simulink model "func2_b"  (R2020a)
settings: Solver=VariableStepAuto  StartTime=0.0  StopTime=10.0  RelTol=1e-3  EnableMultiTasking=on
undefined symbols (not defined in the file or in its folder): S, vsva2197, xcvc1902
libraries: ModelComposer x2, parametrization_2_lib x1
settings Model: Creator=abehbood  LastModifiedBy=viswanad
settings DataIOCC: ReturnWorkspaceOutputs=off
settings OptimizationCC: LifeSpan=inf
settings DebuggingCC: SFUnexpectedBacktrackingDiag=warning  SFNoUnconditionalDefaultTransitionDiag=warning  ArithmeticOperatorsInVariantConditions=warning
settings SFSimCC: SimUseLocalCustomCode=off  CustomCodeUndefinedFunction=UseInterfaceOnly
settings RTWCC: RTWUseLocalCustomCode=off
settings CodeAppCC: StateflowObjectComments=on
settings GRTTargetCC: TargetLangStandard=C89/C90 (ANSI)
settings ConfigComp: CovMetricSettings=dw  CovHtmlReporting=on  CovSaveCumulativeToWorkspaceVar=on  CovSaveSingleToWorkspaceVar=on  CovExternalEMLEnable=off

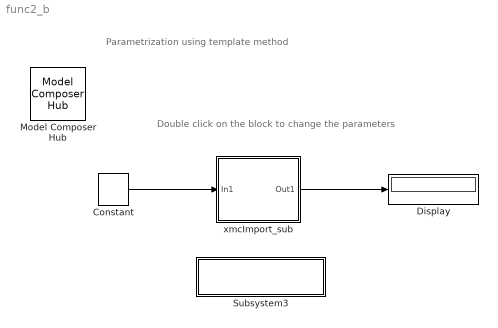
== system func2_b ==
  note: Double click on the block to change the parameters
  note: Parametrization using
      | template method
  Constant : ModelComposer/Constant  Value=1  VectorParams1D=off  SampleTime=1.0  OutDataType=int16  TypeExp=''  Signedness=Signed  WordLength=16  FractionalLength=0  RoundingMode=Truncation to minus infinity  OverflowMode=Wrap around
  Display : Display
  Model Composer Hub : ModelComposer/Model Composer Hub  CodeGeneration=off  SubsystemName=xmcImport_sub  TargetDirectory=./code  ExportType=IP Catalog  IpVendor=xilinx.com  IpLibrary=hls  IpVersion=1.0  IpHWLanguage=Verilog  AieCompilerOptions={}  CreateTestbench=off  TestbenchStackSize=10  RunAieSim=off  AieSimTimeout=50000  RunAieSimProfiling=off  LaunchVitisAnalyzer=off  PlotOutput=off  RunX86Sim=off  X86SimTimeout=10  GenHwImage=off  PlatformType=Not Specified  ProjDevice=xcvc1902-vsva2197-2MP-e-S  ProjDevicePart=xcvc1902-vsva2197-2MP-e-S  SamplePeriod=-1  ClockFrequency=200  DataPathParallelism=1
  Subsystem3 : Subsystem
      settings: OpenFcn=xmcOpenFileEx
      mask Display: disp(sprintf('Double Click to open\nthe main header file'))
  xmcImport_sub : Subsystem
  wires:
  Constant/1 -> xmcImport_sub/1(In1)
  xmcImport_sub/1(Out1) -> Display/1

== system func2_b/Subsystem3 ==

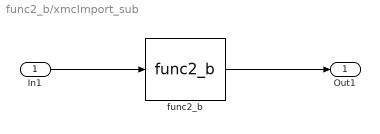
== system func2_b/xmcImport_sub ==
  In1 : Inport
  func2_b : parametrization_2_lib/func2_b  LibraryFunction=func2_b  IncludeFiles={'func2_b.h'}  SourceFiles={}  IncludeDirectories={}  TemplateParams={'int P1'; 'int P2'}  FunctionParamTypes={xmcDataType('void'); xmcDataType('int16_t'); xmcDataType('int8_t &'); xmcDataType('int'); xmcDataType('int')}  FunctionParamPassbys={0.000000000000000000e+00; 0.000000000000000000e+00; 1.000000000000000000e+00; 0.000000000000000000e+00; 0.000000000000000000e+00}  FunctionParamDimensions={'1'; '1'; '1'; '1'; '1'}  FunctionParamNames={'return'; 'in'; 'out'; 'P1'; 'P2'}  FunctionParamDir={0.000000000000000000e+00; 1.000000000000000000e+00; 2.000000000000000000e+00; 3.000000000000000000e+00; 3.000000000000000000e+00}  FunctionParamSupportsStreaming={false; false; false; false; false}  BufferDepth={'0'}  FunctionParamValues={'0'; '0'; '0'; '0'; '0'}  ThroughputFactors={''}  P1=0  P2=0
  Out1 : Outport
  wires:
  In1/1 -> func2_b/1
  func2_b/1 -> Out1/1
